simulink model "AM_Coherent"  (Simulink 6.5)
settings: Solver=FixedStepDiscrete  StartTime=0.0  StopTime=inf  RelTol=1e-3
undefined symbols (not defined in the file or in its folder): bit, dfilt
libraries: c6713dsklib x2, rtdxBlocks x2, dspsrcs4 x2, c6000tgtpreflib x1, dspmathops x1, dspsigops x1, dsparch4 x1, dspindex x1
settings Model: Creator=jfaing  LastModifiedBy=dsp  ProdHWDeviceType=TI C6000
settings SolverCC: PositivePriorityOrder=on
settings DataIOCC: SaveOutput=off  SaveTime=off
settings OptimizationCC: OptimizeModelRefInitCode=on
settings DebuggingCC: MultiTaskDSMMsg=warning  MultiTaskCondExecSysMsg=none
settings HardwareCC: ProdBitPerLong=40  ProdIntDivRoundTo=Zero  ProdEndianess=LittleEndian  ProdHWDeviceType=TI C6000
settings RTWCC: SystemTargetFile=ti_c6000_ert.tlc  GenCodeOnly=on  TemplateMakefile=ti_c6000_ert.tmf  Description=Embedded Target for TI C6000 DSP (ERT)  ProcessScript=ti_c6000_ert_make_rtw_hook  IncludeERTFirstTime=on
settings CodeAppCC: IgnoreCustomStorageClasses=off
settings C6000ERTTargetCC: TargetFcnLib=ansi_tfl_tmw.mat  GenFloatMathFcnCalls=ANSI_C  UtilityFuncGeneration=Auto  GenerateFullHeader=on  GenerateSampleERTMain=off  GenerateTestInterfaces=off  IsPILTarget=off  ModelReferenceCompliant=on  IncludeMdlTerminateFcn=on  CombineOutputUpdateFcns=on  SuppressErrorStatus=off  IncludeFileDelimiter=Auto  ERTCustomFileBanners=on  SupportAbsoluteTime=on  LogVarNameModifier=rt_  MatFileLogging=off  MultiInstanceERTCode=off  SupportNonFinite=on  SupportComplex=on  PurelyIntegerCode=off  SupportContinuousTime=off  SupportNonInlinedSFcns=off  EnableShiftOperators=on  ParenthesesLevel=Nominal  GenerateErtSFunction=off  GenerateASAP2=off  ExtMode=off  ExtModeTransport=0  ExtModeStaticAlloc=off  ExtModeStaticAllocSize=1000000  ExtModeTesting=off  ExtModeMexFile=ext_comm  InlinedParameterPlacement=NonHierarchical  TargetOS=BareBoardExample  MultiInstanceErrorCode=Error  RateGroupingCode=on  RootIOFormat=Individual arguments  RTWCAPISignals=off  RTWCAPIParams=off  RTWCAPIStates=off  ERTSrcFileBannerTemplate=ert_code_template.cgt  ERTHdrFileBannerTemplate=ert_code_template.cgt  ERTDataSrcFileTemplate=ert_code_template.cgt  ERTDataHdrFileTemplate=ert_code_template.cgt  ERTCustomFileTemplate=example_file_process.tlc  ModuleNamingRule=Unspecified  SignalDisplayLevel=10  ParamTuneLevel=10  GlobalDataDefinition=Auto  DataDefinitionFile=global.c  GlobalDataReference=Auto  DataReferenceFile=global.h  GRTInterface=off  EnableUserReplacementTypes=off  MemSecPackage=--- None ---  MemSecDataConstants=Default  MemSecDataIO=Default  MemSecDataInternal=Default  MemSecDataParameters=Default  MemSecFuncInitTerm=Default  MemSecFuncExecute=Default  exportCCSObj=on  ccsObjName=CCS_Obj  useDSPBIOS=on  ProfileGenCode=off  InlineDSPBlks=on  FPopt=off  memModel=Far_Aggregate  optLevel=Function(-o2)  CompilerVerbosity=Quiet  InterruptThreshOnC6x=off  SymbolicDebugOnC6x=off  RetainAsmFiles=off  RetainObjFiles=on  CreateMapFile=on  UserStackSize=8192  c6000BuildAction=Build  OverrunAction=Notify_and_continue  OverrunNotificationMethod=Turn_on_LEDs

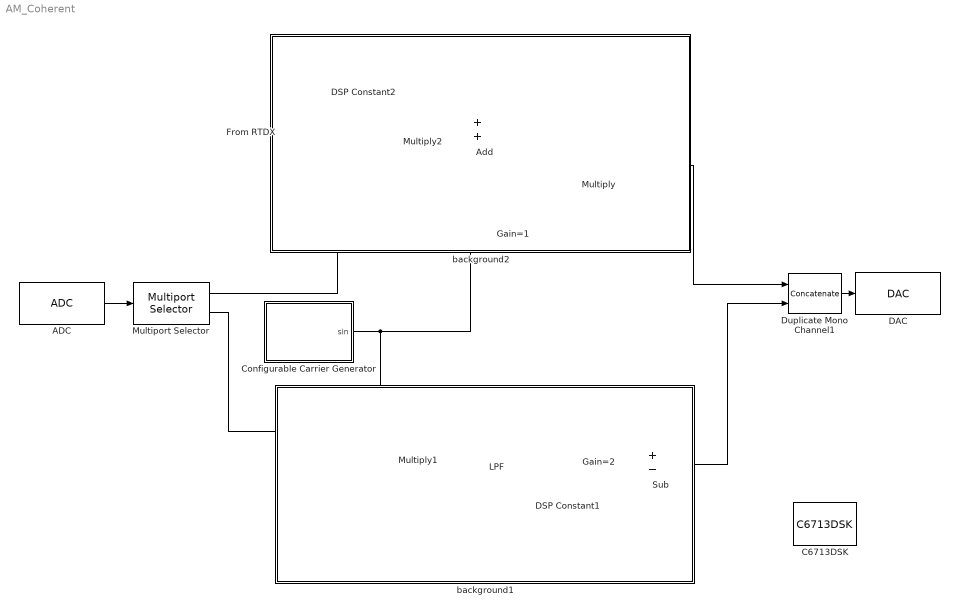
== system AM_Coherent ==
  ADC : c6713dsklib/ADC  ADCsource=Line In  MicGain=off  Stereo=on  SampleRate=96 kHz  CodecDataFormat=16-bit  OutputDataType=Single  Scaling=Normalize  SourceGain=0.0  FrameSize=64  inheritSampleTime=off
  Add : Sum  OutScaling=2^-10
  C6713DSK : c6000tgtpreflib/C6713DSK  Tag=C6000 TARGET PREFERENCES BLOCK  SystemSampleTime=-1
  Configurable Carrier Generator : Subsystem
  DAC : c6713dsklib/DAC  CodecDataFormat=16-bit  SampleRate=96 kHz  Scaling=Normalize  DacAtten=0.0  OverflowMode=Wrap
  DSP Constant1 : dspsrcs4/DSP Constant  SystemSampleTime=-1  Value=0.5  SampleMode=Discrete  discreteOutput=Frame-based  continuousOutput=Sample-based  sampTime=1/96000  framePeriod=-1  dataType=single  isSigned=on  wordLen=16  udDataType=sfix(16)  fracBitsMode=Best precision  numFracBits=15  InterpretAs1D=-inf  Ts=-inf  FramebasedOutput=-inf
  DSP Constant2 : dspsrcs4/DSP Constant  SystemSampleTime=-1  Value=0.5  SampleMode=Discrete  discreteOutput=Frame-based  continuousOutput=Sample-based  sampTime=1/96000  framePeriod=-1  dataType=single  isSigned=on  wordLen=16  udDataType=sfix(16)  fracBitsMode=Best precision  numFracBits=15  InterpretAs1D=-inf  Ts=-inf  FramebasedOutput=-inf
  Duplicate Mono Channel1 : Concatenate  Mode=Horizontal matrix concatenation
  From RTDX : rtdxBlocks/From RTDX  channelNameStr=InputModulation  isBlocking=off  icMaskVar=1  Ts=-1  dims=[1 1]  isFrame=off  dType=single  isChannelEnabled=on  isHighSpeedRTDXUsed=on
  Gain=1 : Gain
  Gain=2 : Gain  Gain=2
  LPF : dsparch4/Digital Filter  Tag=BlockMethodSubSystem  DialogController=dspdialog.DigitalFilter  DialogControllerArgs=DataTag1  TypePopup=FIR (all zeros)  IIRFiltStruct=Direct form II transposed  AllPoleFiltStruct=Direct form  FIRFiltStruct=Direct form  CoeffSource=Specify via dialog  NumCoeffs=[0.000488939681944421 0.00172830941349848 0.00395876781732765 0.00679313323619244 0.00907869940855358 0.00915670414650422 0.0056785418076704 -0.00132324324390355 -0.00975074336536299 -0.0158037730552593 -0.0156105347479998 -0.00756349568140769 0.00588396633058039 0.0182959531627658 0.021796977679317 0.0113171156250792 -0.0114696244186289 -0.0368732393512304 -0.0499720675038943 -0.036861279612986 0.00824101524106748 0.0785398754492806 0.155494554858895 0.21517691742281 0.237647742263117 0.21517691742281 0.155494554858895 0.0785398754492806 0.00824101524106748 -0.036861279612986 -0.0499720675038943 -0.0368732393512304 -0.0114696244186289 0.0113171156250792 0.021796977679317 0.0182959531627658 0.00588396633058039 -0.00756349568140769 -0.0156105347479998 -0.0158037730552593 -0.00975074336536299 -0.00132324324390355 0.0056785418076704 0.00915670414650422 0.00907869940855358 0.00679313323619244 0.00395876781732765 0.00172830941349848 0.000488939681944421]  DenCoeffs=[1 0.1]  BiQuadCoeffs=[1 0.3 0.4 1 0.1 0.2]  LatticeCoeffs=[0.2 0.4]  denIgnore=on  FiltPerSampPopup=One filter per frame  IC=0  ICnum=0  ICden=0  roundingMode=Floor  overflowMode=off  ScaleValues=1  scaleValueFracLength=14  stageInFracLength=15  stageOutFracLength=15  FilterSource=Specify via dialog  dfiltObjectName=dfilt.dffir([1 2 1])
  Multiply : Product  Inputs=**  OutScaling=2^-10  InputSameDT=on
  Multiply1 : Product  Inputs=**  OutScaling=2^-10  InputSameDT=on
  Multiply2 : Product  Inputs=**  OutScaling=2^-10  InputSameDT=on
  Multiport Selector : dspindex/Multiport Selector  rowsOrCols=Columns  idxCellArray={ 1,2 }  idxErrMode=Clip Index
  Sub : Sum  Inputs=+-  OutScaling=2^-10
  background1 : Subsystem
      settings: AttributesFormatString=AM Receiver
      mask Display: disp('')
  background2 : Subsystem
      settings: AttributesFormatString=AM Transmitter
      mask Display: disp('')
  wires:
  Configurable Carrier Generator/1(sin) -> Multiply1/2, Gain=1/1
  Multiply1/1 -> LPF/1
  Gain=1/1 -> Multiply/2
  ADC/1 -> Multiport Selector/1
  Duplicate Mono Channel1/1 -> DAC/1
  Gain=2/1 -> Sub/1
  DSP Constant1/1 -> Sub/2
  Multiport Selector/2 -> Multiply1/1
  Add/1 -> Multiply/1
  Multiport Selector/1 -> Add/2
  LPF/1 -> Gain=2/1
  Sub/1 -> Duplicate Mono Channel1/2
  DSP Constant2/1 -> Multiply2/1
  Multiply2/1 -> Add/1
  From RTDX/1 -> Multiply2/2
  Multiply/1 -> Duplicate Mono Channel1/1

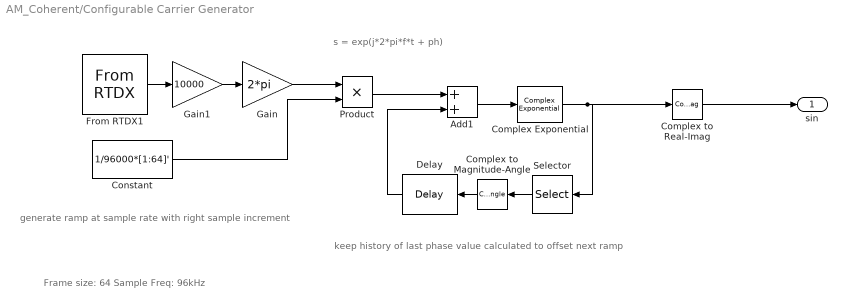
== system AM_Coherent/Configurable Carrier Generator ==
  note: keep history of last phase value calculated
      | to offset next ramp
  note: s = exp(j*2*pi*f*t + ph)
  note: generate ramp at sample rate
      | with right sample increment
  note: Frame size: 64
      | Sample Freq: 96kHz
  Add1 : Sum  OutScaling=2^-10
  Complex Exponential : dspmathops/Complex Exponential  SystemSampleTime=-1
  Complex to Magnitude-Angle : ComplexToMagnitudeAngle  Orientation=left  Output=Angle
  Complex to Real-Imag : ComplexToRealImag  Output=Real
  Constant : Constant  Value=1/96000*[1:64]'  VectorParams1D=off  OutDataTypeMode=single  OutDataType=sfix(16)  ConRadixGroup=Use specified scaling  OutScaling=2^0  SampleTime=0.001  FramePeriod=64/96000
      settings: SamplingMode=Frame based
  Delay : dspsigops/Delay  Orientation=left  dly_unit=Samples  delay=1  ic_detail=off  dif_ic_for_ch=off  dif_ic_for_dly=off  ic=0  reset_popup=None
  From RTDX1 : rtdxBlocks/From RTDX  channelNameStr=freq  isBlocking=off  icMaskVar=1  Ts=-1  dims=[1 1]  isFrame=off  dType=single  isChannelEnabled=on  isHighSpeedRTDXUsed=on
  Gain : Gain  Gain=2*pi
  Gain1 : Gain  Gain=10000
  Product : Product  RndMeth=Zero
  Selector : Selector  Orientation=left  InputType=Vector  ElementSrc=Internal  Elements=[64]  RowSrc=Internal  Rows=1  ColumnSrc=Internal  Columns=1  InputPortWidth=64  IndexIsStartValue=off
  sin : Outport
  wires:
  Gain1/1 -> Gain/1
  Complex to Real-Imag/1 -> sin/1
  Add1/1 -> Complex Exponential/1
  Product/1 -> Add1/1
  Delay/1 -> Add1/2
  Complex to Magnitude-Angle/1 -> Delay/1
  Selector/1 -> Complex to Magnitude-Angle/1
  Complex Exponential/1 -> Selector/1, Complex to Real-Imag/1
  Gain/1 -> Product/1
  Constant/1 -> Product/2
  From RTDX1/1 -> Gain1/1

== system AM_Coherent/background1 ==

== system AM_Coherent/background2 ==
